simulink model "SingleHold_Model"  (R2025a)
settings: Solver=VariableStepAuto  StartTime=0.0  StopTime=10.0  RelTol=1e-3
libraries: NSA_DEVS_SINKS x4, NSA_DEVS_SOURCES x2, NSA_DEVS_LOGISTICS x1
settings Model: Creator=david  LastModifiedBy=peter
settings RTWCC: GPUComputeCapability=3.5

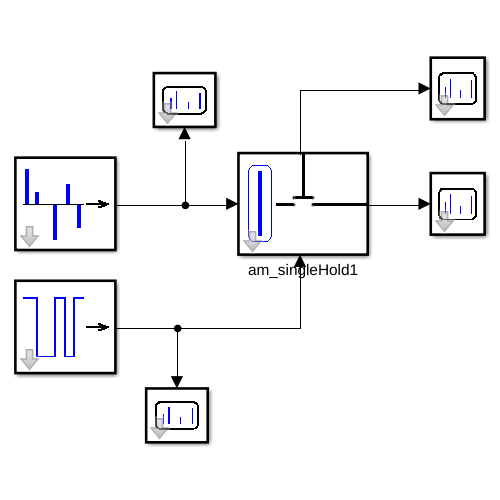
[thumbnail: Simulink's stored preview of the top-level diagram]
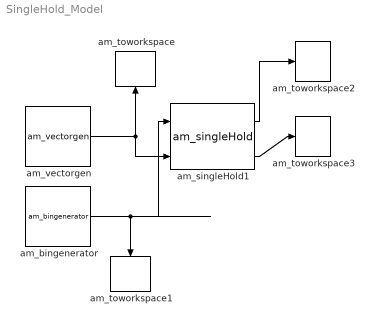
== system SingleHold_Model ==
  am_bingenerator : NSA_DEVS_SOURCES/am_bingenerator  z0=false  tVec=[2.0, 2.1, 3.5, 3.6, 5.5, 7.5, 12.0, 12.1, 15.0, 15.1, 16.0, 16.1,100]  tau=[0,1]  debug=0
      settings: SourceProductName=Sources
  am_singleHold1 : NSA_DEVS_LOGISTICS/am_singleHold  tau=[0,1]  debug=0
      settings: SourceProductName=Logistics
  am_toworkspace : NSA_DEVS_SINKS/am_toworkspace  varname="\"inE\""  t0=0  format="\"vector\""  tau=[0,5]  debug=0
      settings: SourceProductName=Sinks
  am_toworkspace1 : NSA_DEVS_SINKS/am_toworkspace  varname="\"inCond\""  t0=0  format="\"vector\""  tau=[0,5]  debug=0
      settings: SourceProductName=Sinks
  am_toworkspace2 : NSA_DEVS_SINKS/am_toworkspace  varname="\"outDrop\""  t0=0  format="\"vector\""  tau=[0,5]  debug=0
      settings: SourceProductName=Sinks
  am_toworkspace3 : NSA_DEVS_SINKS/am_toworkspace  varname="\"outE\""  t0=0  format="\"vector\""  tau=[0,5]  debug=0
      settings: SourceProductName=Sinks
  am_vectorgen : NSA_DEVS_SOURCES/am_vectorgen  tvec=[1 3 5 7 9 11 13 15 100]  yvec=[1 2 1 2 1 2 1 2 1]  tau=[0,1]  debug=0
      settings: SourceProductName=Sources
  wires:
  am_singleHold1/1 -> am_toworkspace3/1
  am_vectorgen/1 -> am_singleHold1/1, am_toworkspace/1
  am_bingenerator/1 -> am_singleHold1/2, am_toworkspace1/1
  am_singleHold1/2 -> am_toworkspace2/1
